simulink model "simulink_traverse"  (R2021b)
settings: Solver=ode45  StartTime=0.0  StopTime=20  RelTol=1e-3
values from neighbouring files (symbols this model uses):
  ts3 = 10^-3    (= 0.001)    [loading_project.m]
libraries: simulink x3
settings Model: Creator=noait  LastModifiedBy=noait

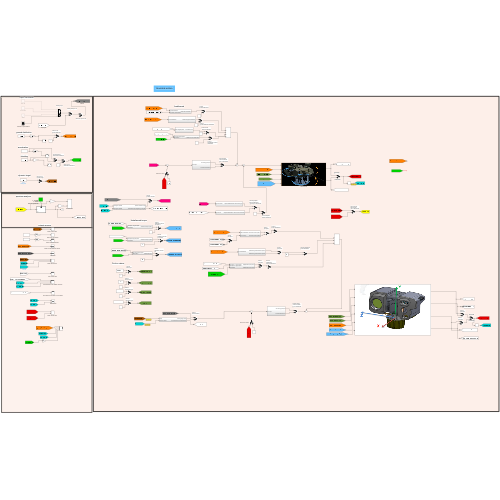
[thumbnail: Simulink's stored preview of the top-level diagram]
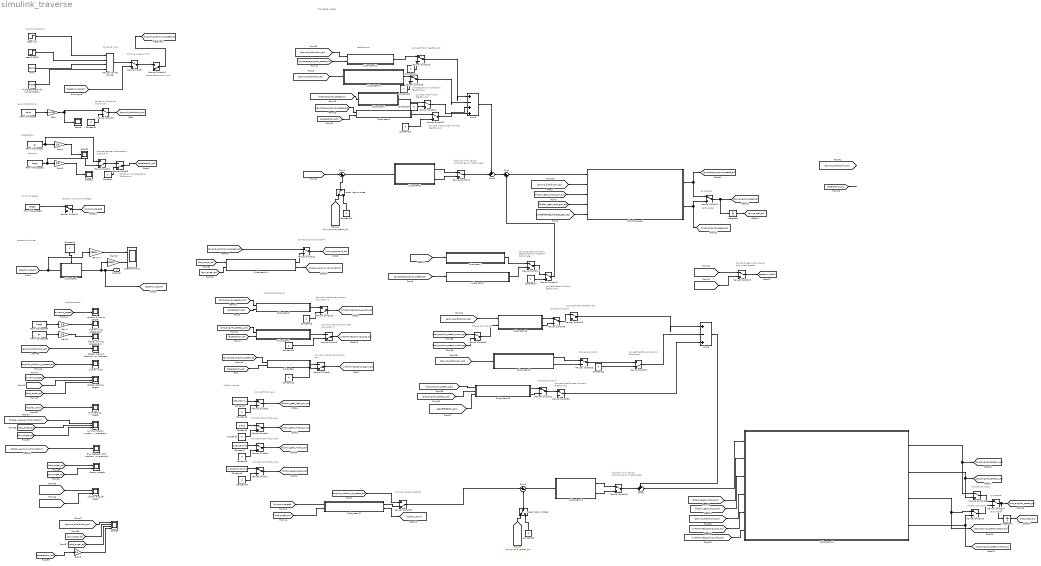
== system simulink_traverse ==
  note: TRAVERSE MODEL
  note: connect motor
      |  friction feedforward
  note: feedforward
  note: spectrum analyzer
  note: dynamic target
  note: acceleration
  note: ground distribution
  note: shooting
  note: input:Time domain
  note: Friction values
  note: Unballanced torque
  note: tachometer
  note: gyroscope
  note: cancel or not
      | synamic target
  note: cancel or not
      | acceleration distribution
  note: choose between
      | acceleration distribution
  note: cancel or not
      | ground distribution
  note: choosing input
  note: chosing sweep or not
  note: disconnect input or not
  note: connect
      | ground distribution feedforward
  note: connect
      | friction feedforward
  note: connect
      | unballanced moment
      | feedforward
  note: chossing setpoint
      | friction feedforward
      |  gyroscope or tachometer
  note: connect setpoint
      | friction feedforward
  note: choose sweep
      | output signal
      |  pod or tachometer
  note: choose
      | pod option
  note: choose
      | pod option
  note: choose
      | pod option
  note: choose
      | pod option
  note: choose
      | pod option
  note: choose
      | pod option
  note: gyroscope
  note: tachometer
  note: chossing which
      |  sensor controller
      | gyro or tachometer
  note: chossing which
      |  sensor controller
      | gyro or tachometer
  note: connect
      | friction gun
  note: connect
      | motor friction-gun
  note: connect
      | motor friction-pod
  note: connect
      | load friction-pod
  note: connect
      | unballance moment
      | gun
  note: connect
      | unballance moment
      | pod option 2
  note: connect
      | unballance moment
      | pod option 1
  note: connect
      | position controller
  note: connect feedforward
      | ground distribution
  note: connect
      | friction feedforward
  note: connect
      | unballanced
      | moment feedforward
  note: connect
      | inertia controller
  note: outputs scopes
  " plant traverse4" : Subsystem
      mask Display: image('C:\Users\noait\OneDrive\Desktop\צילום.png'); % Use "Edit Image" on toolstrip to change.
  " synchronization system stability accuaracy" : Scope  NumInputPorts=3
  Constant : Constant  Value=0  SampleTime=-1
  Constant1 : Constant  OutDataTypeStr=boolean
      settings: AttributesFormatString=1 - START\n0 -STOP\ninternal spectrum
      settings: OpenFcn=|
      | if get_param(gcbh,'value')-48 set_param(gcbh,'value','0','backgroundcolor','red');
      | else set_param(gcbh,'value','1','backgroundcolor','green');
      | end
  Constant{4,6,8,10..20,22} (15 alike) : Constant  Value=0  SampleTime=0
  Constant2 : Constant  Value=0  SampleTime=-1
  Constant3 : Constant  Value=0.021  SampleTime=0
  Constant5 : Constant  Value=1300/(200*1.1)  SampleTime=0
  Constant7 : Constant  Value=0.23125*0.42  SampleTime=0
  Constant9 : Constant  Value=0.23125*0.42*0.5  SampleTime=0
  Error between pod position to gun position1 : Scope
  From Workspace : FromWorkspace  VariableName=trdist  SampleTime=ts3/3  Interpolate=off  ZeroCross=off  OutputAfterFinalValue=Setting to zero
  From Workspace1 : FromWorkspace  VariableName=gy  SampleTime=ts3/3  Interpolate=off  ZeroCross=off  OutputAfterFinalValue=Setting to zero
  From Workspace2 : FromWorkspace  VariableName=firegy  SampleTime=ts3/9  Interpolate=off  ZeroCross=off  OutputAfterFinalValue=Setting to zero
  From Workspace3 : FromWorkspace  VariableName=targetx  SampleTime=5*ts3  Interpolate=off  ZeroCross=off  OutputAfterFinalValue=Setting to zero
  From Workspace4 : FromWorkspace  VariableName=firegz  SampleTime=ts3/9  Interpolate=off  ZeroCross=off  OutputAfterFinalValue=Setting to zero
  From Workspace5 : FromWorkspace  VariableName=gz  SampleTime=ts3/3  Interpolate=off  ZeroCross=off  OutputAfterFinalValue=Setting to zero
  Gain : Gain  Gain=pi/180
  Gain{1..5} (5 alike) : Gain  Gain=9.8
  Gain17 : Gain  Gain=180/pi
  Gain18 : Gain  Gain=180/pi
  Integrator : Integrator  ZeroCross=off
  Integrator1 : Integrator  ZeroCross=off
  Manual Variant Source : simulink/Signal Routing/Manual Variant Source  NumChoices=4  LabelModeActiveChoice=V_4
  Manual Switch{,3..7,11..15,17..26,28..32,34} (27 alike) : ManualSwitch
  Manual Switch{1..2,8..10,16,27,33} (8 alike) : ManualSwitch  CurrentSetting=0
  Pulse Generator for syncronization : DiscretePulseGenerator  PulseType=Time based  Period=10  PulseWidth=50
  Scope : Scope
  Scope1 : Scope
  Scope2 : Scope
  Scope3 : Scope  NumInputPorts=4
  SpectrumInOut : Scope  NumInputPorts=2
  Step 1[A] : Step  SampleTime=0  ZeroCross=off
  Subsystem : Subsystem
  Subsystem1 : Subsystem  mask{GAIN=0.22%2*pi/180%0.5*pi/180, InitFreq=1, TargetTime=500, FreqAtTime=500}
      mask prompts: InitFreq "INITIAL FREQUENCY"; TargetTime "Target Time"; FreqAtTime "Frequency at Time"
  Subsystem10 : Subsystem
  Subsystem11 : Subsystem
      mask Display: image('C:\Users\noait\OneDrive\Desktop\צילום מסך 2024-04-08 195106.png'); % Use "Edit Image" on toolstrip to change.
  Subsystem12 : Subsystem
  Subsystem13 : Subsystem
  Subsystem14 : Subsystem
  Subsystem15 : Subsystem
  Subsystem16 : Subsystem
  Subsystem17 : Subsystem
  Subsystem2 : Subsystem
  Subsystem3 : Subsystem
  Subsystem4 : Subsystem
  Subsystem5 : Subsystem
  Subsystem6 : Subsystem
  Subsystem7 : Subsystem
  Subsystem8 : Subsystem
  Subsystem9 : Subsystem
  Sum : Sum  Inputs=|++
  Sum1 : Sum  Inputs=|+-
  Sum2 : Sum  Inputs=++|
  Sum3 : Sum  Inputs=|+-++
  Sum4 : Sum  Inputs=|+-
  Sum5 : Sum  Inputs=++|
  Sum6 : Sum  Inputs=|+-+
  display angels : Scope  NumInputPorts=2
  display angular speed : Scope  NumInputPorts=2
  display driving acceleration : Scope
  display dynamic target : Scope
  display firing acceleration : Scope
  display ground distribution [rad/sec] : Scope
  display input : Scope
  display tracking target : Scope  NumInputPorts=3
  error tracking target : Scope
  open loop or close : ManualSwitch
  open loop or close1 : ManualSwitch
  ramp : simulink/Sources/Ramp  slope=1  start=0  InitialOutput=0
  step 0.05[A] : Step  After=0.05  SampleTime=0  ZeroCross=off
  Output2 : Outport
  wires:
  Pulse Generator for syncronization/1 -> Manual Variant Source/4
  Manual Switch/1 -> Manual Switch16/1
  Manual Switch2/1 -> [acceleration_az]
  Manual Switch1/1 -> Manual Switch2/1
  From Workspace2/1 -> Manual Switch1/2, Gain2/1
  Manual Switch16/1 -> [angular_position_or_speed_az]
  Constant2/1 -> Manual Switch3/2
  Gain1/1 -> Scope1/1
  Gain/1 -> Manual Switch3/1, Scope/1
  Manual Switch3/1 -> [ground_distribution_az]
  Gain2/1 -> Scope2/1
  Constant/1 -> Manual Switch2/2
  Manual Variant Source/1 -> Manual Switch/1
  Step 1[A]/1 -> Manual Variant Source/1
  From Workspace1/1 -> Manual Switch1/1, Gain1/1
  step 0.05[A]/1 -> Manual Variant Source/2
  ramp/1 -> Manual Variant Source/3
  From Workspace/1 -> Gain/1
  [spectrum_signal] -> Manual Switch/2
  Manual Switch4/1 -> [friction_gear_motor_gun_az]
  Constant6/1 -> Manual Switch5/2
  Manual Switch5/1 -> [friction_gear_load_gun_az]
  Constant10/1 -> Manual Switch7/2
  Constant8/1 -> Manual Switch6/2
  Constant4/1 -> Manual Switch4/2
  Manual Switch7/1 -> [friction_gear_load_pod]
  Manual Switch6/1 -> [friction_gear_motor_pod]
  Constant5/1 -> Manual Switch5/1
  Constant7/1 -> Manual Switch6/1
  Constant9/1 -> Manual Switch7/1
  Constant3/1 -> Manual Switch4/1
  [gyroscope_angular_speed_az] -> Subsystem/1(gyroscope angular speed)
  [acceleration_az] -> Subsystem/2(acceleration)
  [acceleration_az] -> Subsystem2/2(acceleration)
  Subsystem2/1(unballanced torque option2) -> Manual Switch9/1
  Constant11/1 -> Manual Switch8/2
  Subsystem/1(unballanced torque) -> Manual Switch8/1
  Manual Switch10/1 -> [unballanced_torque_pod1_az]
  [acceleration_az] -> Subsystem3/2(acceleration)
  Manual Switch8/1 -> [unballanced_torque_gun_az]
  Manual Switch9/1 -> [unballanced_torque_pod2_az]
  Subsystem3/1(unballanced torque option1) -> Manual Switch10/1
  Constant13/1 -> Manual Switch10/2
  [pod_angular_speed_2_az] -> Subsystem2/1(pod option2 angular speed)
  Constant12/1 -> Manual Switch9/2
  [pod_angular_speed_1_az] -> Subsystem3/1("pod option1  angular speed ")
  [ground_distribution_az] -> " plant traverse4"/2(external distribution)
  [friction_gear_load_gun_az] -> " plant traverse4"/4(load friction az value)
  [friction_gear_motor_gun_az] -> " plant traverse4"/3(motor friction value az)
  [unballanced_torque_gun_az] -> " plant traverse4"/5(unballanced torque az)
  Integrator/1 -> [gun_angel_az]
  Manual Switch12/1 -> Integrator/1, [gun_angular_speed_az]
  " plant traverse4"/1(gun speed gyroscope) -> [gyroscope_angular_speed_az], Manual Switch12/1
  " plant traverse4"/2(motor speed tachometer) -> [motor_angular_speed_az], Manual Switch12/2
  Gain17/1 -> SpectrumInOut/1
  Gain18/1 -> SpectrumInOut/2
  [spectrum_back] -> Gain17/1, Subsystem1/1(Input)
  Subsystem1/1(Output2) -> [spectrum_signal], Output2/1, Gain18/1
  Constant1/1 -> Subsystem1/Enable
  Manual Switch25/1 -> [spectrum_back]
  [gun_angular_speed_az] -> Manual Switch25/1
  [pod_angular_speed_az] -> Manual Switch25/2
  Subsystem5/2(out control tachometer) -> Manual Switch13/2
  Subsystem5/1(out control gyroscope) -> Manual Switch13/1
  Sum1/1 -> Subsystem5/1(error input)
  Constant14/1 -> open loop or close/2
  [gun_angular_speed_az] -> open loop or close/1
  open loop or close/1 -> Sum1/2
  [input_command_az] -> Sum1/1
  Manual Switch11/1 -> [input_command_az]
  Sum/1 -> " plant traverse4"/1(current command traverse)
  Sum2/1 -> Sum/1
  [gyroscope_angular_speed_az] -> Subsystem4/1(gyroscope angular speed)
  [acceleration_az] -> Subsystem4/2(acceleration)
  Manual Switch13/1 -> Sum2/2
  Sum3/1 -> Sum2/1
  Manual Switch21/1 -> Sum3/3
  Subsystem4/1(unballanced torque feedforward) -> Manual Switch21/1
  Constant15/1 -> Manual Switch21/2
  Subsystem7/1(setpoint feedforward for reduce friction gyro) -> Manual Switch17/1
  [gyroscope_angular_speed_az] -> Subsystem8/1(gyro sensor)
  [motor_angular_speed_az] -> Subsystem6/1(motor angular speed)
  Constant16/1 -> Manual Switch14/2
  Subsystem6/1(anti friction motor) -> Manual Switch14/1
  Manual Switch14/1 -> Sum3/4
  Manual Switch17/1 -> Manual Switch18/1
  Subsystem8/1(setpoint feedforward for reduce friction tachometer) -> Manual Switch17/2
  Manual Switch18/1 -> Sum/2
  Constant17/1 -> Manual Switch18/2
  Constant18/1 -> Manual Switch15/2
  Subsystem9/1(feedforward ground distribution) -> Manual Switch15/1
  [ground_distribution_az] -> Subsystem9/1(ground distribution)
  [ground_distribution_az] -> Subsystem10/1(ground distribution)
  Constant19/1 -> Manual Switch19/2
  Subsystem10/1(feedforward load friction) -> Manual Switch19/1
  Manual Switch19/1 -> Sum3/1
  Manual Switch15/1 -> Sum3/2
  [gyroscope_angular_speed_az] -> Subsystem10/2(gyroscope angular speed)
  [friction_gear_motor_pod] -> Subsystem11/2(motor torque value pod)
  [friction_gear_load_pod] -> Subsystem11/3(torque load value pod)
  [ground_distribution_az] -> Subsystem11/4(external distribution)
  [unballanced_torque_pod1_az] -> Subsystem11/5(unballanced torque option1)
  [unballanced_torque_pod2_az] -> Subsystem11/6(unballanced torque option 2)
  Manual Switch23/1 -> Manual Switch24/2
  Subsystem11/3(tachometer motor angular speed option 1) -> [pod_angular_speed_motor1_az], Manual Switch23/1
  Subsystem11/4(tachometer motor angular speed option2) -> [pod_angular_speed_motor2_az], Manual Switch23/2
  Subsystem11/2(gyroscope output option2) -> Manual Switch22/2, [pod_angular_speed_2_az]
  Manual Switch24/1 -> Integrator1/1, [pod_angular_speed_az]
  Integrator1/1 -> [pod_angel_az]
  Subsystem11/1(gyroscope output option 1) -> Manual Switch22/1, [pod_angular_speed_1_az]
  Manual Switch22/1 -> Manual Switch24/1
  [pod_angular_speed_az] -> open loop or close1/1
  Constant20/1 -> open loop or close1/2
  open loop or close1/1 -> Sum4/2
  Sum4/1 -> Subsystem12/1(error input)
  Subsystem12/1(out control gyroscope) -> Manual Switch20/1
  Subsystem12/2(out control tachometer) -> Manual Switch20/2
  Manual Switch20/1 -> Sum5/2
  Sum5/1 -> Subsystem11/1(input current)
  [ground_distribution_az] -> Subsystem13/1(ground distribution)
  Constant22/1 -> Manual Switch27/2
  Manual Switch27/1 -> Sum6/2
  Subsystem13/1(feedforward ground distribution option1) -> Manual Switch26/1
  Subsystem13/2(feedforward ground distribution option2) -> Manual Switch26/2
  Manual Switch26/1 -> Manual Switch27/1
  Sum6/1 -> Sum5/1
  Manual Switch28/1 -> Sum6/1
  Subsystem16/2(unballanced torque option2) -> Manual Switch31/2
  Manual Switch30/1 -> Manual Switch28/1
  [pod_angular_speed_motor2_az] -> Manual Switch29/2
  [pod_angular_speed_2_az] -> Subsystem16/2("pod option2  angular speed ")
  Subsystem15/1(anti friction current option1) -> Manual Switch30/1
  Subsystem15/2(anti friction current option2) -> Manual Switch30/2
  Subsystem16/1(unballanced torque option1) -> Manual Switch31/1
  Manual Switch31/1 -> Manual Switch32/1
  [pod_angular_speed_1_az] -> Subsystem16/1("pod option1  angular speed ")
  [acceleration_az] -> Subsystem16/3(acceleration)
  [ground_distribution_az] -> Subsystem15/1(external distribution)
  [pod_angular_speed_motor1_az] -> Manual Switch29/1
  Manual Switch29/1 -> Subsystem15/2(motor velocity)
  Manual Switch32/1 -> Sum6/3
  [gun_angel_az] -> Subsystem14/2(gun angular position)
  Subsystem14/1(position controller output) -> Manual Switch11/2
  [pod_angel_az] -> Subsystem14/1(pod angular position)
  [angular_position_or_speed_az] -> Manual Switch11/1
  [input_command_az] -> Subsystem7/1(gyro command)
  [pod_angel_az] -> Subsystem17/2(pod gun position)
  Subsystem17/1(error targeting control) -> Manual Switch33/2
  [angular_position_or_speed_az] -> Manual Switch33/1
  Manual Switch33/1 -> Sum4/1
  [acceleration_az] -> ?
  Manual Switch34/1 -> [dynamic_target]
  From Workspace3/1 -> Manual Switch34/1
  [dynamic_target] -> Subsystem17/1(target)
  [gun_angel_az] -> " synchronization system stability accuaracy"/3
  [ground_distribution_az] -> display ground distribution [rad/sec]/1
  [gun_angular_speed_az] -> display angular speed/1
  [gun_angel_az] -> display angels/2
  Gain5/1 -> display driving acceleration/1
  From Workspace5/1 -> Gain5/1
  [dynamic_target] -> display dynamic target/1
  [pod_angel_az] -> display tracking target/3
  [pod_angel_az] -> Scope3/3
  [display_error_synchronization] -> " synchronization system stability accuaracy"/1
  [display_error_synchronization] -> Error between pod position to gun position1/1
  [pod_angel_az] -> display angels/1
  [gun_angel_az] -> display tracking target/2
  [acceleration_az] -> Gain3/1
  From Workspace4/1 -> Gain4/1
  Gain4/1 -> display firing acceleration/1
  [ground_distribution_az] -> Scope3/1
  Gain3/1 -> Scope3/4
  [angular_position_or_speed_az] -> display input/1
  [pod_angular_speed_az] -> display angular speed/2
  [pod_angel_az] -> " synchronization system stability accuaracy"/2
  [gun_angel_az] -> Scope3/2
  [dynamic_target] -> display tracking target/1
  [display_error] -> error tracking target/1
  Subsystem17/2(error between target to pod position) -> [display_error]
  Subsystem14/2(Error between pod angular to gun angular) -> [display_error_synchronization]

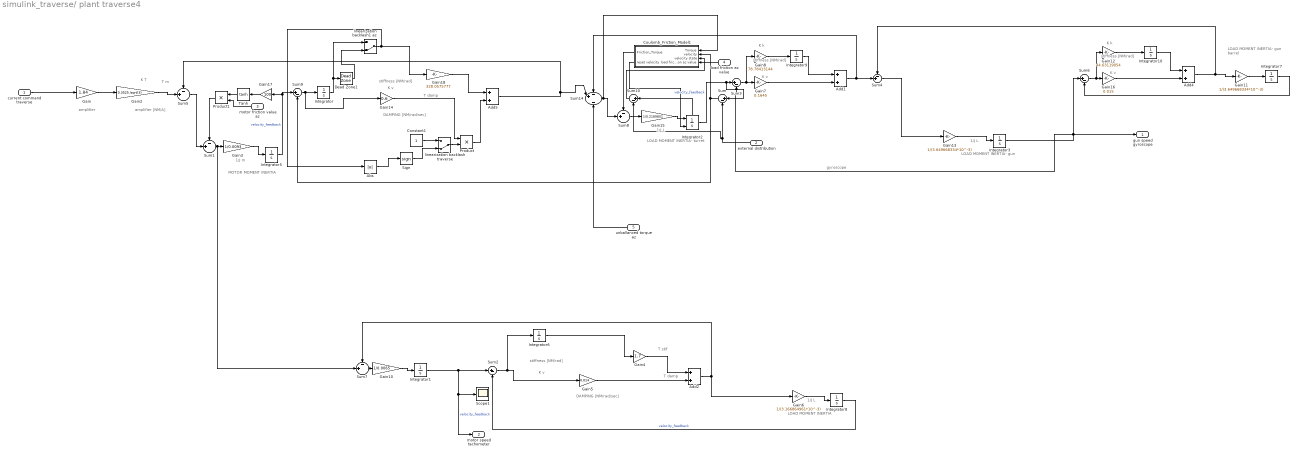
== system simulink_traverse/ plant traverse4 ==
  note: gyroscope
  note: K v
  note: T m
  note: stiffness
      | [NM/rad]
  note: K T
  note: K k
  note: MOTOR
      | MOMENT INERTIA
  note: amplifier
      | [NM/A]
  note: 1/J m
  note: K v
  note: stiffness
      | [NM/rad]
  note: K k
  note: LOAD
      | MOMENT INERTIA- gun
  note: 1/J L
  note: 1/J L
  note: stiffness
      | [NM/rad]
  note: T damp
  note: DAMPING
      | [NM/rad/sec]
  note: LOAD
      | MOMENT INERTIA
  note: K v
  note: T stif
  note: stiffness
      | [NM/rad]
  note: T damp
  note: DAMPING
      | [NM/rad/sec]
  note: LOAD
      | MOMENT INERTIA- turret
  note: K v
  note: 1/J L
  note: LOAD
      | MOMENT INERTIA- gun barrel
  note: amplifier
  current command traverse : Inport
  external distribution : Inport  Port=2
  motor friction value az : Inport  Port=3
  load friction az value : Inport  Port=4
  unballanced torque az : Inport  Port=5
  Abs : Abs
  Add{1..2,4..5} (4 alike) : Sum
  Constant1 : Constant
  Coulomb_Friction_Model1 : Subsystem
  Dead Zone1 : DeadZone  LowerValue=-0.07*10^-3  UpperValue=0.07*10^-3  ZeroCross=off
  Gain : Gain  Gain=1.84
  Gain10 : Gain  Gain=1/0.0065
  Gain11 : Gain  Gain=1/(3.649668334*10^-3)
  Gain12 : Gain  Gain=44.63119054
  Gain13 : Gain  Gain=1/(3.649668334*10^-3)
  Gain14 : Gain  Gain=0.6
  Gain15 : Gain  Gain=1/0.2189801
  Gain16 : Gain  Gain=0.015
  Gain17 : Gain  Gain=100
  Gain18 : Gain  Gain=328.0575777
  Gain2 : Gain  Gain=0.3525 /sqrt(3)
  Gain3 : Gain  Gain=1/0.0093
  Gain4 : Gain  Gain=1.7
  Gain5 : Gain  Gain=0.014
  Gain6 : Gain  Gain=1/(3.166864961*10^-3)
  Gain7 : Gain  Gain=0.1645
  Gain8 : Gain  Gain=78.78413144
  Integrator{,6..7,9..10} (5 alike) : Integrator
  Integrator{1,3,5,8} (4 alike) : Integrator  ZeroCross=off
  Integrator2 : Integrator  ExternalReset=rising  ShowStatePort=on  ZeroCross=off
  Product : Product
  Product1 : Product
  Scope1 : Scope
  Sign : Signum
  Sum{,2..3,6,9..10} (6 alike) : Sum  Inputs=|+-
  Sum1 : Sum  Inputs=-+|  SaturateOnIntegerOverflow=on
  Sum14 : Sum  Inputs=-+|-  SaturateOnIntegerOverflow=on
  Sum4 : Sum  Inputs=-+|
  Sum5 : Sum  Inputs=-+|
  Sum7 : Sum  Inputs=-+|  SaturateOnIntegerOverflow=on
  Sum8 : Sum  Inputs=-+|  SaturateOnIntegerOverflow=on
  Tanh : Trigonometry  Operator=tanh
  linearization backlash traverse : ManualSwitch  CurrentSetting=0
  linearization backlash1 az : ManualSwitch  CurrentSetting=0
  gun speed gyroscope : Outport
  motor speed tachometer : Outport  Port=2
  wires:
  Gain12/1 -> Integrator10/1
  Sum5/1 -> Sum1/2
  Integrator7/1 -> Sum6/2
  Gain/1 -> Gain2/1
  Integrator9/1 -> Add1/1
  Gain3/1 -> Integrator5/1
  Gain16/1 -> Add4/2
  Add1/1 -> Sum4/2, Sum14/1
  Gain6/1 -> Integrator8/1
  Gain14/1 -> Product/1
  Gain2/1 -> Sum5/2
  Sum3/1 -> Gain7/1, Gain8/1
  Gain7/1 -> Add1/2
  Gain10/1 -> Integrator1/1
  Gain11/1 -> Integrator7/1
  Gain8/1 -> Integrator9/1
  Integrator8/1 -> Sum2/2  "velocity_feedback"
  Integrator3/1 -> gun speed gyroscope/1, Sum3/2, Sum6/1
  Sum2/1 -> Integrator6/1, Gain5/1
  Sum4/1 -> Gain13/1
  Add4/1 -> Gain11/1, Sum4/1
  Integrator10/1 -> Add4/1
  Integrator2/1 -> Sum/1, Sum3/1  "velocity_feedback"
  Sum9/1 -> Gain14/1, Integrator/1
  Sum6/1 -> Gain16/1, Gain12/1
  Gain15/1 -> Integrator2/1
  Sum7/1 -> Gain10/1
  Add2/1 -> Gain6/1, Sum7/1
  Sum1/1 -> Sum7/2, Gain3/1
  Integrator5/1 -> Sum9/1, Gain17/1  "velocity_feedback"
  Add5/1 -> Sum5/1, Sum14/2
  Gain13/1 -> Integrator3/1
  Integrator1/1 -> motor speed tachometer/1, Scope1/1, Sum2/1  "velocity_feedback"
  current command traverse/1 -> Gain/1
  Sign/1 -> linearization backlash traverse/2
  Abs/1 -> Sign/1
  linearization backlash traverse/1 -> Product/2
  Constant1/1 -> linearization backlash traverse/1
  Product/1 -> Add5/2
  Dead Zone1/1 -> linearization backlash1 az/2
  Integrator/1 -> linearization backlash1 az/1, Dead Zone1/1
  linearization backlash1 az/1 -> Abs/1, Gain18/1
  Gain18/1 -> Add5/1
  Gain4/1 -> Add2/1
  Gain5/1 -> Add2/2
  Integrator6/1 -> Gain4/1
  Sum8/1 -> Gain15/1
  Sum14/1 -> Coulomb_Friction_Model1/1(Torque), Sum8/2
  Coulomb_Friction_Model1/1(Friction_Torque) -> Sum8/1
  Coulomb_Friction_Model1/2(reset velocity) -> Integrator2/2
  Sum/1 -> Coulomb_Friction_Model1/2(velocity), Sum9/2
  Sum10/1 -> Coulomb_Friction_Model1/3(velocity state)
  external distribution/1 -> Sum10/2, Sum/2
  Integrator2/State -> Sum10/1
  Gain17/1 -> Tanh/1
  Tanh/1 -> Product1/1
  Product1/1 -> Sum1/1
  motor friction value az/1 -> Product1/2
  load friction az value/1 -> Coulomb_Friction_Model1/4(load friction az value)
  unballanced torque az/1 -> Sum14/3

== system simulink_traverse/Subsystem ==
  gyroscope angular speed : Inport
  acceleration : Inport  Port=2
  Cos2 : Trigonometry
  Gain1 : Gain  Gain=4866/200
  Gain2 : Gain  Gain=4866/200
  Integrator : Integrator  ZeroCross=off
  Sum : Sum  Inputs=|++
  unballanced torque : Outport
  wires:
  Integrator/1 -> Cos2/1
  gyroscope angular speed/1 -> Integrator/1
  Cos2/1 -> Gain2/1
  acceleration/1 -> Gain1/1
  Sum/1 -> unballanced torque/1
  Gain1/1 -> Sum/2
  Gain2/1 -> Sum/1

== system simulink_traverse/Subsystem1 ==
  Input : Inport
  Enable : EnablePort  StatesWhenEnabling=reset
  Chirp Signal1 : simulink/Sources/Chirp Signal  f1=1  T=160  f2=160
  Mux2 : Mux  Inputs=2
  Scope2 : Scope
  TSABAD_out_log : Scope
  gain 3 : Gain  Gain=GAIN  SaturateOnIntegerOverflow=on  SampleTime=ts3  OutDataTypeStr=Inherit: Same as input  ParamDataTypeStr=Inherit: Same as input
  Output2 : Outport
  wires:
  gain 3/1 -> Output2/1, Mux2/1
  Input/1 -> Mux2/2
  Mux2/1 -> TSABAD_out_log/1
  Chirp Signal1/1 -> gain 3/1, Scope2/1

== system simulink_traverse/Subsystem10 ==
  ground distribution : Inport
  gyroscope angular speed : Inport  Port=2
  Gain : Gain  Gain=-1
  Gain14 : Gain  Gain=sqrt(3)/0.3525
  Gain15 : Gain  Gain=1300/(200*1.1)
  Gain16 : Gain  Gain=1/1.84
  Gain19 : Gain  Gain=100
  Sum : Sum  Inputs=|++
  Tanh : Trigonometry  Operator=tanh
  Transfer Fcn1 : TransferFcn  Numerator=[0.02219 1.182 1026 1.42*10^4 5.857*10^6]  Denominator="[0.003183 2.538  528.2 3.284*10^4 5.857*10^6]"
  feedforward load friction : Outport
  wires:
  Gain19/1 -> Tanh/1
  Tanh/1 -> Gain15/1
  Gain15/1 -> Gain16/1
  Gain16/1 -> Gain14/1
  Gain14/1 -> feedforward load friction/1
  ground distribution/1 -> Gain/1
  gyroscope angular speed/1 -> Transfer Fcn1/1
  Gain/1 -> Sum/1
  Sum/1 -> Gain19/1
  Transfer Fcn1/1 -> Sum/2

== system simulink_traverse/Subsystem11 ==
  input current : Inport
  motor torque value pod : Inport  Port=2
  torque load value pod : Inport  Port=3
  external distribution : Inport  Port=4
  unballanced torque option1 : Inport  Port=5
  unballanced torque option 2 : Inport  Port=6
  Subsystem : Subsystem
  Subsystem1 : Subsystem
  gyroscope output option 1 : Outport
  gyroscope output option2 : Outport  Port=2
  tachometer motor angular speed option 1 : Outport  Port=3
  tachometer motor angular speed option2 : Outport  Port=4
  wires:
  Subsystem/1(tachometer motor angular speed option1) -> tachometer motor angular speed option 1/1
  Subsystem/2(gyroscope output option1) -> gyroscope output option 1/1
  Subsystem1/1(tachometer motor angular speed option2) -> tachometer motor angular speed option2/1
  Subsystem1/2(gyroscope output option2) -> gyroscope output option2/1
  motor torque value pod/1 -> Subsystem1/2(motor torque value pod), Subsystem/2(motor torque value pod)
  torque load value pod/1 -> Subsystem/3(torque load value pod), Subsystem1/3(torque load value pod)
  external distribution/1 -> Subsystem1/4(external distribution), Subsystem/4(external distribution)
  unballanced torque option1/1 -> Subsystem/5(unballanced torque option1)
  unballanced torque option 2/1 -> Subsystem1/5(unballanced torque option 2)
  input current/1 -> Subsystem1/1(Input current), Subsystem/1(Input current)

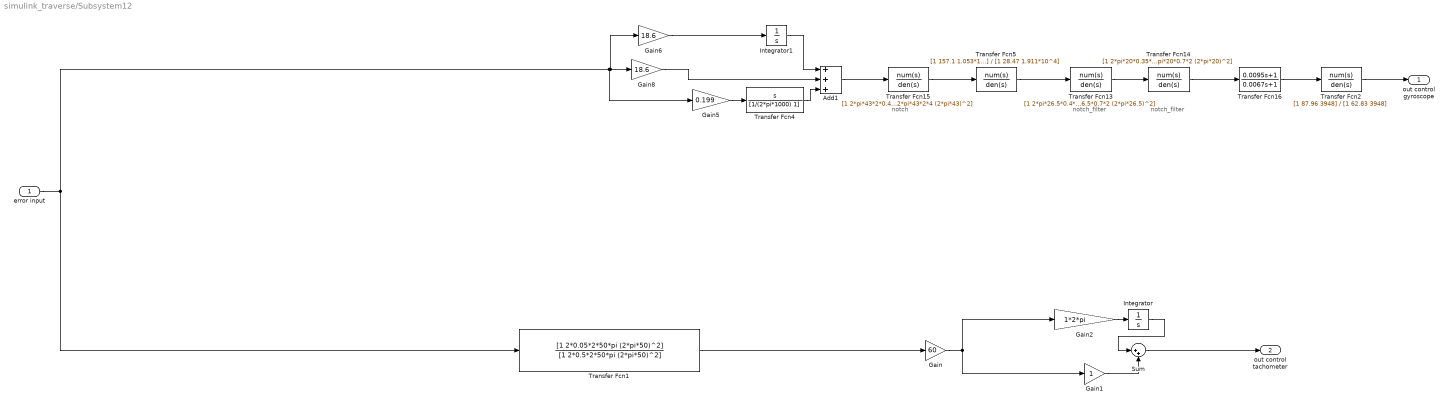
== system simulink_traverse/Subsystem12 ==
  note: notch_filter
  note: notch_filter
  note: notch
  error input : Inport
  Add1 : Sum  Inputs=+++
  Gain : Gain  Gain=60
  Gain1 : Gain
  Gain2 : Gain  Gain=1*2*pi
  Gain5 : Gain  Gain=0.199
  Gain6 : Gain  Gain=18.6
  Gain8 : Gain  Gain=18.6
  Integrator : Integrator
  Integrator1 : Integrator
  Sum : Sum  Inputs=|++
  Transfer Fcn1 : TransferFcn  Numerator=[1 2*0.05*2*50*pi (2*pi*50)^2]  Denominator=[1 2*0.5*2*50*pi (2*pi*50)^2]
  Transfer Fcn13 : TransferFcn  Numerator=[1 2*pi*26.5*0.4*2 (2*pi*26.5)^2]  Denominator=[1 2*pi*26.5*0.7*2 (2*pi*26.5)^2]
  Transfer Fcn14 : TransferFcn  Numerator=[1 2*pi*20*0.35*2 (2*pi*20)^2]  Denominator=[1 2*pi*20*0.7*2 (2*pi*20)^2]
  Transfer Fcn15 : TransferFcn  Numerator="[1 2*pi*43*2*0.4  (2*pi*43)^2]"  Denominator=[1 2*pi*43*2*4 (2*pi*43)^2]
  Transfer Fcn16 : TransferFcn  Numerator=[0.0095 1]  Denominator=[0.0067 1]
  Transfer Fcn2 : TransferFcn  Numerator=[1 87.96 3948]  Denominator=[1 62.83 3948]
  Transfer Fcn4 : TransferFcn  Numerator=[1 0]  Denominator=[1/(2*pi*1000) 1]
  Transfer Fcn5 : TransferFcn  Numerator=[1 157.1 1.053*10^5]  Denominator=[1 28.47 1.911*10^4]
  out control gyroscope : Outport
  out control tachometer : Outport  Port=2
  wires:
  Gain1/1 -> Sum/2
  Gain2/1 -> Integrator/1
  Integrator/1 -> Sum/1
  Gain/1 -> Gain1/1, Gain2/1
  Sum/1 -> out control tachometer/1
  Transfer Fcn1/1 -> Gain/1
  error input/1 -> Transfer Fcn1/1, Gain5/1, Gain6/1, Gain8/1
  Transfer Fcn5/1 -> Transfer Fcn13/1
  Transfer Fcn14/1 -> Transfer Fcn16/1
  Transfer Fcn13/1 -> Transfer Fcn14/1
  Gain5/1 -> Transfer Fcn4/1
  Integrator1/1 -> Add1/1
  Transfer Fcn15/1 -> Transfer Fcn5/1
  Gain6/1 -> Integrator1/1
  Gain8/1 -> Add1/2
  Add1/1 -> Transfer Fcn15/1
  Transfer Fcn4/1 -> Add1/3
  Transfer Fcn16/1 -> Transfer Fcn2/1
  Transfer Fcn2/1 -> out control gyroscope/1

== system simulink_traverse/Subsystem13 ==
  ground distribution : Inport
  Gain1 : Gain  Gain=1/1.4833
  Gain10 : Gain  Gain=1/1.47
  Gain8 : Gain  Gain=0.015
  Gain9 : Gain  Gain=1/1.057
  Transfer Fcn1 : TransferFcn  Numerator=[1 0]  Denominator=[1/(2*pi*1000) 1]
  feedforward ground distribution option1 : Outport
  feedforward ground distribution option2 : Outport  Port=2
  wires:
  Transfer Fcn1/1 -> Gain8/1
  Gain8/1 -> Gain9/1
  Gain9/1 -> Gain1/1, Gain10/1
  ground distribution/1 -> Transfer Fcn1/1
  Gain1/1 -> feedforward ground distribution option2/1
  Gain10/1 -> feedforward ground distribution option1/1

== system simulink_traverse/Subsystem14 ==
  pod angular position : Inport
  gun angular position : Inport  Port=2
  Gain : Gain  Gain=15.5
  Gain1 : Gain
  Gain2 : Gain  Gain=0.8
  Integrator : Integrator  ZeroCross=off
  Sum : Sum  Inputs=|+-
  Sum1 : Sum  Inputs=|+++
  Transfer Fcn : TransferFcn  Numerator=[1 0]  Denominator=[1/(2*pi*100) 1]
  position controller output : Outport
  Error between pod angular to gun angular : Outport  Port=2
  wires:
  pod angular position/1 -> Sum/1
  gun angular position/1 -> Sum/2
  Sum/1 -> Gain2/1, Error between pod angular to gun angular/1, Gain/1
  Sum1/1 -> position controller output/1
  Gain/1 -> Sum1/2, Gain1/1
  Gain1/1 -> Integrator/1
  Integrator/1 -> Sum1/1
  Gain2/1 -> Transfer Fcn/1
  Transfer Fcn/1 -> Sum1/3

== system simulink_traverse/Subsystem15 ==
  external distribution : Inport
  motor velocity : Inport  Port=2
  Gain2 : Gain  Gain=0.23125*0.42*0.5
  Gain21 : Gain  Gain=1/1.057
  Gain23 : Gain  Gain=1/1.483
  Gain3 : Gain  Gain=-1
  Gain4 : Gain  Gain=100
  Gain41 : Gain  Gain=1/1.47
  Gain6 : Gain  Gain=100
  Gain7 : Gain  Gain=0.23125*0.42
  Sum : Sum  Inputs=|++
  Tanh : Trigonometry  Operator=tanh
  Tanh1 : Trigonometry  Operator=tanh
  anti friction current option1 : Outport
  anti friction current option2 : Outport  Port=2
  wires:
  external distribution/1 -> Gain3/1
  Gain3/1 -> Gain4/1
  Gain4/1 -> Tanh/1
  Tanh/1 -> Gain2/1
  Tanh1/1 -> Gain7/1
  Gain6/1 -> Tanh1/1
  motor velocity/1 -> Gain6/1
  Gain7/1 -> Sum/2
  Gain2/1 -> Sum/1
  Sum/1 -> Gain21/1
  Gain41/1 -> anti friction current option1/1
  Gain21/1 -> Gain23/1, Gain41/1
  Gain23/1 -> anti friction current option2/1

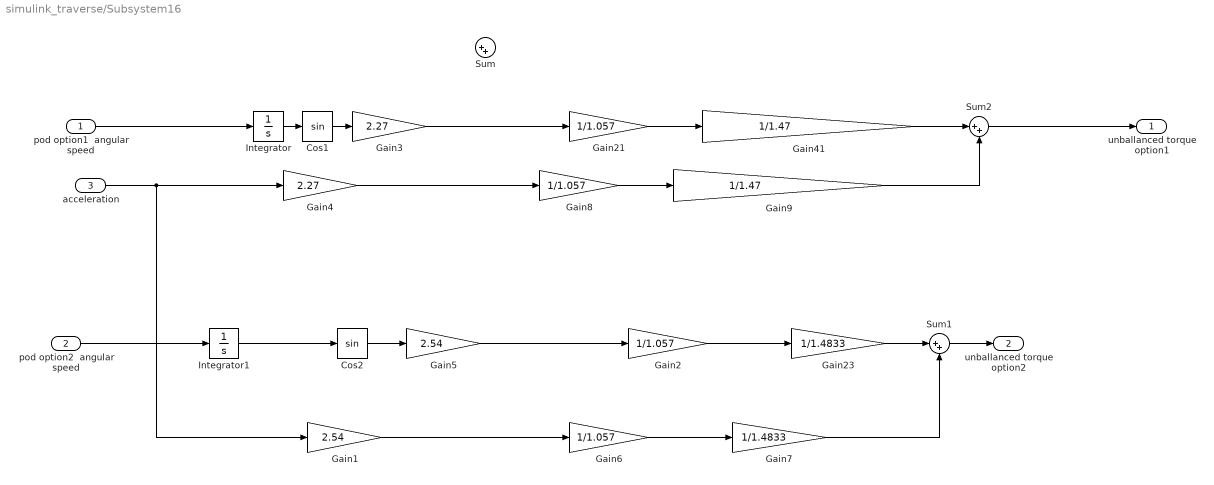
== system simulink_traverse/Subsystem16 ==
  "pod option1  angular speed " : Inport
  "pod option2  angular speed " : Inport  Port=2
  acceleration : Inport  Port=3
  Cos1 : Trigonometry
  Cos2 : Trigonometry
  Gain1 : Gain  Gain=2.54
  Gain{2,6,8,21} (4 alike) : Gain  Gain=1/1.057
  Gain23 : Gain  Gain=1/1.4833
  Gain3 : Gain  Gain=2.27
  Gain4 : Gain  Gain=2.27
  Gain41 : Gain  Gain=1/1.47
  Gain5 : Gain  Gain=2.54
  Gain7 : Gain  Gain=1/1.4833
  Gain9 : Gain  Gain=1/1.47
  Integrator : Integrator  ZeroCross=off
  Integrator1 : Integrator  ZeroCross=off
  Sum : Sum  Inputs=|++
  Sum1 : Sum  Inputs=|++
  Sum2 : Sum  Inputs=|++
  unballanced torque option1 : Outport
  unballanced torque option2 : Outport  Port=2
  wires:
  Integrator/1 -> Cos1/1
  acceleration/1 -> Gain1/1, Gain4/1
  "pod option1  angular speed "/1 -> Integrator/1
  Gain21/1 -> Gain41/1
  Integrator1/1 -> Cos2/1
  "pod option2  angular speed "/1 -> Integrator1/1
  Gain2/1 -> Gain23/1
  Cos1/1 -> Gain3/1
  Gain5/1 -> Gain2/1
  Cos2/1 -> Gain5/1
  Gain23/1 -> Sum1/1
  Sum1/1 -> unballanced torque option2/1
  Gain6/1 -> Gain7/1
  Gain1/1 -> Gain6/1
  Gain7/1 -> Sum1/2
  Gain3/1 -> Gain21/1
  Gain41/1 -> Sum2/1
  Sum2/1 -> unballanced torque option1/1
  Gain8/1 -> Gain9/1
  Gain4/1 -> Gain8/1
  Gain9/1 -> Sum2/2

== system simulink_traverse/Subsystem17 ==
  target : Inport
  pod gun position : Inport  Port=2
  Gain : Gain  Gain=30
  Gain1 : Gain  Gain=30
  Gain2 : Gain  Gain=-0.05
  Integrator2 : Integrator
  Sum : Sum  Inputs=|+-
  Sum1 : Sum  Inputs=|+++
  Transfer Fcn : TransferFcn  Numerator=[1 0]  Denominator=[1/(2*pi*1000) 1]
  error targeting control : Outport
  error between target to pod position : Outport  Port=2
  wires:
  target/1 -> Sum/1
  pod gun position/1 -> Gain2/1, Sum/2
  Integrator2/1 -> Sum1/1
  Gain/1 -> Integrator2/1
  Gain2/1 -> Transfer Fcn/1
  Transfer Fcn/1 -> Sum1/3
  Gain1/1 -> Sum1/2
  Sum1/1 -> error targeting control/1
  Sum/1 -> error between target to pod position/1, Gain/1, Gain1/1

== system simulink_traverse/Subsystem2 ==
  pod option2 angular speed : Inport
  acceleration : Inport  Port=2
  Cos1 : Trigonometry
  Gain1 : Gain  Gain=2.54
  Gain3 : Gain  Gain=2.54
  Integrator : Integrator  ZeroCross=off
  Sum : Sum  Inputs=|++
  unballanced torque option2 : Outport
  wires:
  Cos1/1 -> Gain3/1
  pod option2 angular speed/1 -> Integrator/1
  Integrator/1 -> Cos1/1
  Gain3/1 -> Sum/1
  Sum/1 -> unballanced torque option2/1
  acceleration/1 -> Gain1/1
  Gain1/1 -> Sum/2

== system simulink_traverse/Subsystem3 ==
  "pod option1  angular speed " : Inport
  acceleration : Inport  Port=2
  Cos1 : Trigonometry
  Gain1 : Gain  Gain=2.27
  Gain3 : Gain  Gain=2.27
  Integrator : Integrator  ZeroCross=off
  Sum : Sum  Inputs=|++
  unballanced torque option1 : Outport
  wires:
  Cos1/1 -> Gain3/1
  Integrator/1 -> Cos1/1
  "pod option1  angular speed "/1 -> Integrator/1
  acceleration/1 -> Gain1/1
  Gain1/1 -> Sum/2
  Gain3/1 -> Sum/1
  Sum/1 -> unballanced torque option1/1

== system simulink_traverse/Subsystem4 ==
  gyroscope angular speed : Inport
  acceleration : Inport  Port=2
  Cos2 : Trigonometry
  Gain1 : Gain  Gain=4866/200
  Gain2 : Gain  Gain=4866/200
  Gain6 : Gain  Gain=1/1.84
  Gain7 : Gain  Gain=sqrt(3)/0.3525
  Integrator : Integrator  ZeroCross=off
  Sum : Sum  Inputs=|++
  Transfer Fcn : TransferFcn  Numerator=[0.04139 2.67 1460]  Denominator=[1.5292*10^-5 1.078 546.8]
  unballanced torque feedforward : Outport
  wires:
  Integrator/1 -> Cos2/1
  gyroscope angular speed/1 -> Integrator/1
  Cos2/1 -> Gain2/1
  acceleration/1 -> Gain1/1
  Gain6/1 -> Gain7/1
  Sum/1 -> unballanced torque feedforward/1
  Gain2/1 -> Gain6/1
  Gain7/1 -> Sum/1
  Gain1/1 -> Transfer Fcn/1
  Transfer Fcn/1 -> Sum/2

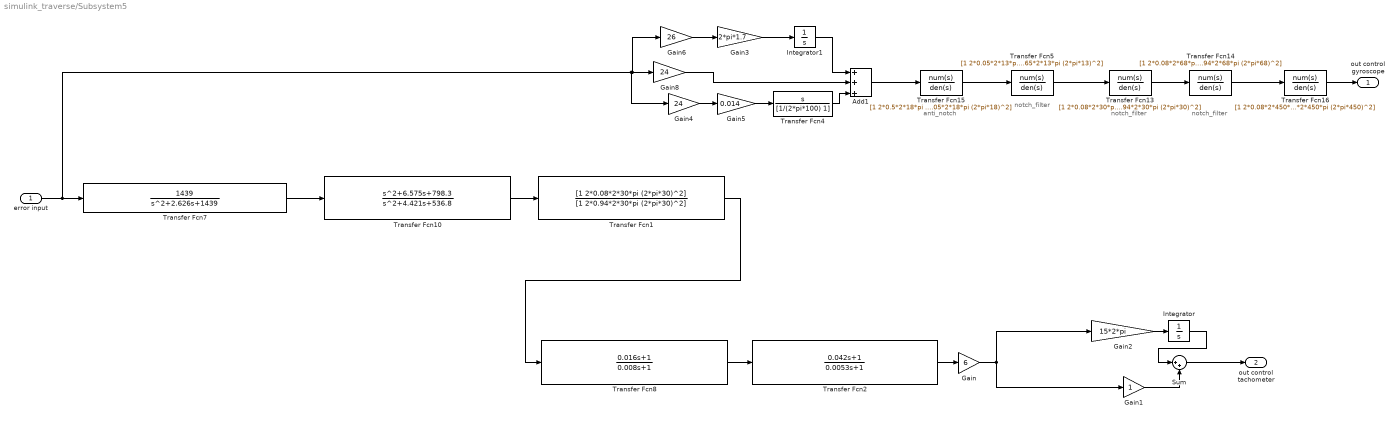
== system simulink_traverse/Subsystem5 ==
  note: notch_filter
  note: notch_filter
  note: notch_filter
  note: anti_notch
  error input : Inport
  Add1 : Sum  Inputs=+++
  Gain : Gain  Gain=6
  Gain1 : Gain
  Gain2 : Gain  Gain=15*2*pi
  Gain3 : Gain  Gain=2*pi*1.7
  Gain4 : Gain  Gain=24
  Gain5 : Gain  Gain=0.014
  Gain6 : Gain  Gain=26
  Gain8 : Gain  Gain=24
  Integrator : Integrator
  Integrator1 : Integrator
  Sum : Sum  Inputs=|++
  Transfer Fcn1 : TransferFcn  Numerator=[1 2*0.08*2*30*pi (2*pi*30)^2]  Denominator=[1 2*0.94*2*30*pi (2*pi*30)^2]
  Transfer Fcn10 : TransferFcn  Numerator=[1 6.575 798.3]  Denominator=[1 4.421 536.8]
  Transfer Fcn13 : TransferFcn  Numerator=[1 2*0.08*2*30*pi (2*pi*30)^2]  Denominator=[1 2*0.94*2*30*pi (2*pi*30)^2]
  Transfer Fcn14 : TransferFcn  Numerator=[1 2*0.08*2*68*pi (2*pi*68)^2]  Denominator=[1 2*0.94*2*68*pi (2*pi*68)^2]
  Transfer Fcn15 : TransferFcn  Numerator=[1 2*0.5*2*18*pi (2*pi*18)^2]  Denominator=[1 2*0.05*2*18*pi (2*pi*18)^2]
  Transfer Fcn16 : TransferFcn  Numerator=[1 2*0.08*2*450*pi (2*pi*450)^2]  Denominator=[1 2*0.94*2*450*pi (2*pi*450)^2]
  Transfer Fcn2 : TransferFcn  Numerator=[0.042 1]  Denominator=[0.0053 1]
  Transfer Fcn4 : TransferFcn  Numerator=[1 0]  Denominator=[1/(2*pi*100) 1]
  Transfer Fcn5 : TransferFcn  Numerator=[1 2*0.05*2*13*pi (2*pi*13)^2]  Denominator=[1 2*0.65*2*13*pi (2*pi*13)^2]
  Transfer Fcn7 : TransferFcn  Numerator=[1439]  Denominator=[1 2.626 1439]
  Transfer Fcn8 : TransferFcn  Numerator=[0.016 1]  Denominator=[0.008 1]
  out control gyroscope : Outport
  out control tachometer : Outport  Port=2
  wires:
  Gain1/1 -> Sum/2
  Transfer Fcn10/1 -> Transfer Fcn1/1
  Transfer Fcn1/1 -> Transfer Fcn8/1
  Gain2/1 -> Integrator/1
  Integrator/1 -> Sum/1
  Gain/1 -> Gain1/1, Gain2/1
  Sum/1 -> out control tachometer/1
  Transfer Fcn7/1 -> Transfer Fcn10/1
  Transfer Fcn8/1 -> Transfer Fcn2/1
  Transfer Fcn2/1 -> Gain/1
  Gain4/1 -> Gain5/1
  Transfer Fcn5/1 -> Transfer Fcn13/1
  error input/1 -> Gain4/1, Gain6/1, Gain8/1, Transfer Fcn7/1
  Transfer Fcn16/1 -> out control gyroscope/1
  Transfer Fcn14/1 -> Transfer Fcn16/1
  Transfer Fcn13/1 -> Transfer Fcn14/1
  Gain5/1 -> Transfer Fcn4/1
  Integrator1/1 -> Add1/1
  Transfer Fcn15/1 -> Transfer Fcn5/1
  Gain3/1 -> Integrator1/1
  Gain8/1 -> Add1/2
  Add1/1 -> Transfer Fcn15/1
  Gain6/1 -> Gain3/1
  Transfer Fcn4/1 -> Add1/3

== system simulink_traverse/Subsystem6 ==
  motor angular speed : Inport
  Gain3 : Gain  Gain=100
  Gain4 : Gain  Gain=0.021
  Gain6 : Gain  Gain=1/1.84
  Gain7 : Gain  Gain=sqrt(3)/0.3525
  Tanh : Trigonometry  Operator=tanh
  Transfer Fcn : TransferFcn  Numerator=[0.6989 4.595 558]  Denominator=[1 4.421 536.8]
  anti friction motor : Outport
  wires:
  Transfer Fcn/1 -> Gain3/1
  Tanh/1 -> Gain4/1
  Gain3/1 -> Tanh/1
  Gain6/1 -> Gain7/1
  Gain4/1 -> Gain6/1
  motor angular speed/1 -> Transfer Fcn/1
  Gain7/1 -> anti friction motor/1

== system simulink_traverse/Subsystem7 ==
  gyro command : Inport
  Gain : Gain  Gain=100
  Gain4 : Gain  Gain=1300/(200*1.1)
  Tanh : Trigonometry  Operator=tanh
  Transfer Fcn1 : TransferFcn  Numerator=[0.04139 2.26 1460]  Denominator=[0.0001592 1.078 546.8]
  Transfer Fcn2 : TransferFcn  Numerator=[0.02219 1.182 1026 1.42*10^4 5.857*10^6]  Denominator="[0.003183 2.538  528.2 3.284*10^4 5.857*10^6]"
  setpoint feedforward for reduce friction gyro : Outport
  wires:
  Gain/1 -> Tanh/1
  Transfer Fcn1/1 -> setpoint feedforward for reduce friction gyro/1
  Gain4/1 -> Transfer Fcn1/1
  Tanh/1 -> Gain4/1
  Transfer Fcn2/1 -> Gain/1
  gyro command/1 -> Transfer Fcn2/1

== system simulink_traverse/Subsystem8 ==
  gyro sensor : Inport
  Gain : Gain  Gain=100
  Gain1 : Gain  Gain=1300/(200*1.1)
  Tanh : Trigonometry  Operator=tanh
  Transfer Fcn : TransferFcn  Numerator=[7.317 4391 5.515*10^5 1.896*10^8 4.492*10^9 1.056*10^12]  Denominator=[1 56.78 4.824*10^4 8.677*10^5 3.438*10^8 1.682*10^9 3.955*10^11]
  Transfer Fcn1 : TransferFcn  Numerator=[0.02219 1.182 1026 1.42*10^4 5.857*10^6]  Denominator=[0.003183 2.538 528.2 3.284*10^4 5.857*10^6]
  setpoint feedforward for reduce friction tachometer : Outport
  wires:
  Gain/1 -> Tanh/1
  Tanh/1 -> Gain1/1
  Gain1/1 -> Transfer Fcn/1
  Transfer Fcn/1 -> setpoint feedforward for reduce friction tachometer/1
  Transfer Fcn1/1 -> Gain/1
  gyro sensor/1 -> Transfer Fcn1/1

== system simulink_traverse/Subsystem9 ==
  ground distribution : Inport
  Gain10 : Gain  Gain=sqrt(3)/0.3525
  Gain8 : Gain  Gain=0.0093
  Gain9 : Gain  Gain=1/1.84
  Transfer Fcn1 : TransferFcn  Numerator=[1 0]  Denominator=[1/(2*pi*100) 1]
  feedforward ground distribution : Outport
  wires:
  Transfer Fcn1/1 -> Gain8/1
  Gain8/1 -> Gain9/1
  Gain9/1 -> Gain10/1
  ground distribution/1 -> Transfer Fcn1/1
  Gain10/1 -> feedforward ground distribution/1

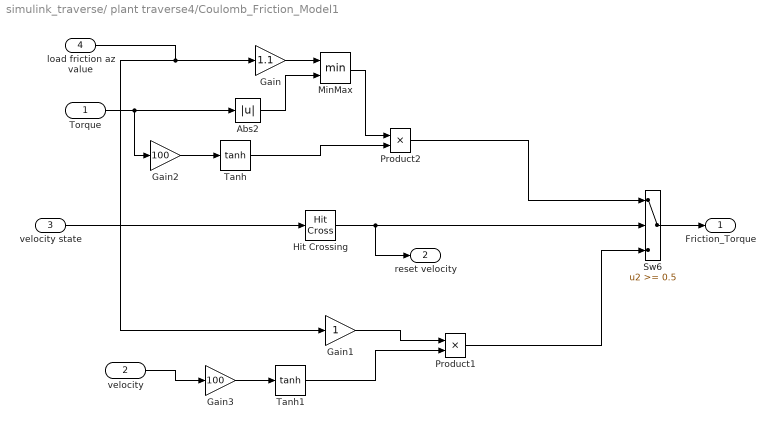
== system simulink_traverse/ plant traverse4/Coulomb_Friction_Model1 ==
  Torque : Inport
  velocity : Inport  Port=2
  velocity state : Inport  Port=3
  load friction az value : Inport  Port=4
  Abs2 : Abs  ZeroCross=off
  Gain : Gain  Gain=1.1
  Gain1 : Gain
  Gain2 : Gain  Gain=100
  Gain3 : Gain  Gain=100
  Hit Crossing : HitCross  ZeroCross=off
  MinMax : MinMax  Inputs=2
  Product1 : Product  RndMeth=Zero
  Product2 : Product  RndMeth=Zero
  Sw6 : Switch  Threshold=0.5  ZeroCross=off  SaturateOnIntegerOverflow=on  InputSameDT=on
  Tanh : Trigonometry  Operator=tanh
  Tanh1 : Trigonometry  Operator=tanh
  Friction_Torque : Outport
  reset velocity : Outport  Port=2
  wires:
  Torque/1 -> Gain2/1, Abs2/1
  Hit Crossing/1 -> reset velocity/1, Sw6/2
  Abs2/1 -> MinMax/2
  MinMax/1 -> Product2/1
  Product2/1 -> Sw6/1
  Product1/1 -> Sw6/3
  velocity state/1 -> Hit Crossing/1
  Gain/1 -> MinMax/1
  Gain1/1 -> Product1/1
  Gain2/1 -> Tanh/1
  Tanh/1 -> Product2/2
  Gain3/1 -> Tanh1/1
  Tanh1/1 -> Product1/2
  velocity/1 -> Gain3/1
  load friction az value/1 -> Gain/1, Gain1/1
  Sw6/1 -> Friction_Torque/1

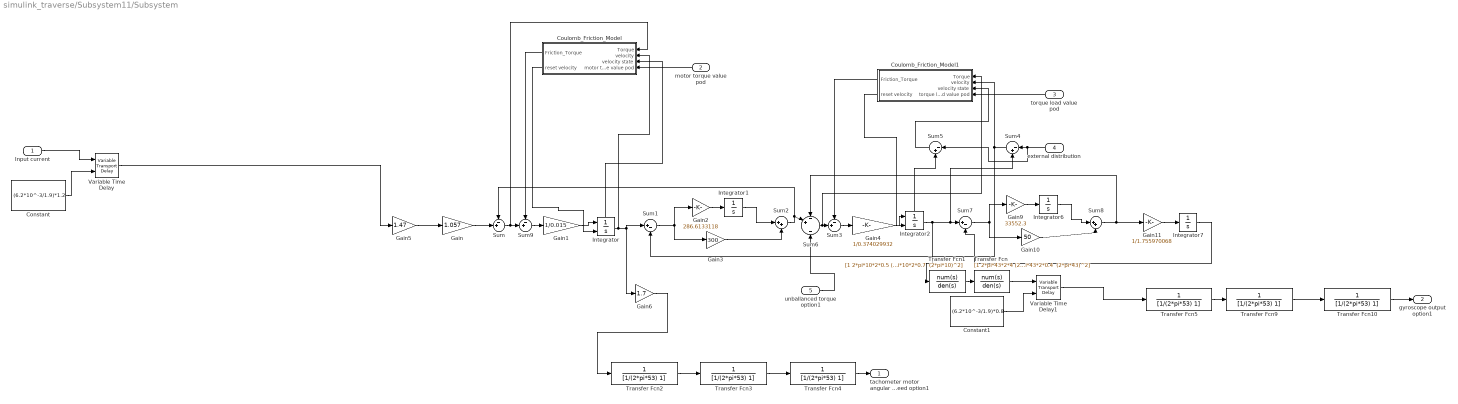
== system simulink_traverse/Subsystem11/Subsystem ==
  Input current : Inport
  motor torque value pod : Inport  Port=2
  torque load value pod : Inport  Port=3
  external distribution : Inport  Port=4
  unballanced torque option1 : Inport  Port=5
  Constant : Constant  Value=(6.2*10^-3/1.9)*1.2  SampleTime=-1
  Constant1 : Constant  Value=(6.2*10^-3/1.9)*0.8  SampleTime=-1
  Coulomb_Friction_Model : Subsystem
  Coulomb_Friction_Model1 : Subsystem
  Gain : Gain  Gain=1.057
  Gain1 : Gain  Gain=1/0.015
  Gain10 : Gain  Gain=50
  Gain11 : Gain  Gain=1/1.755970068
  Gain2 : Gain  Gain=286.6133118
  Gain3 : Gain  Gain=300
  Gain4 : Gain  Gain=1/0.374029932
  Gain5 : Gain  Gain=1.47
  Gain6 : Gain  Gain=1.7
  Gain9 : Gain  Gain=33552.3
  Integrator : Integrator  ExternalReset=rising  ShowStatePort=on  ZeroCross=off
  Integrator1 : Integrator
  Integrator2 : Integrator  ExternalReset=rising  ShowStatePort=on  ZeroCross=off
  Integrator6 : Integrator
  Integrator7 : Integrator
  Sum : Sum  Inputs=-+|
  Sum1 : Sum  Inputs=|+-
  Sum2 : Sum  Inputs=|++
  Sum3 : Sum  Inputs=-+|
  Sum4 : Sum  Inputs=|-+
  Sum5 : Sum  Inputs=|-+
  Sum6 : Sum  Inputs=-+|-
  Sum7 : Sum  Inputs=|+-
  Sum8 : Sum  Inputs=|++
  Sum9 : Sum  Inputs=-+|
  Transfer Fcn : TransferFcn  Numerator=[1 2*pi*43*2*4 (2*pi*43)^2]  Denominator="[1 2*pi*43*2*0.4  (2*pi*43)^2]"
  Transfer Fcn1 : TransferFcn  Numerator=[1 2*pi*10*2*0.5 (2*pi*10)^2]  Denominator="[1 2*pi*10*2*0.7  (2*pi*10)^2]"
  Transfer Fcn{2..5,9..10} (6 alike) : TransferFcn  Denominator=[1/(2*pi*53) 1]
  Variable Time Delay : VariableTransportDelay  MaximumDelay=10  TransDelayFeedthrough=on
  Variable Time Delay1 : VariableTransportDelay  MaximumDelay=10  TransDelayFeedthrough=on
  tachometer motor angular speed option1 : Outport
  gyroscope output option1 : Outport  Port=2
  wires:
  Sum1/1 -> Gain3/1, Gain2/1
  Transfer Fcn/1 -> Variable Time Delay1/1
  Constant1/1 -> Variable Time Delay1/2
  Variable Time Delay/1 -> Gain5/1
  Gain1/1 -> Integrator/1
  Sum8/1 -> Gain11/1, Sum6/1
  Gain11/1 -> Integrator7/1
  Input current/1 -> Variable Time Delay/1
  Integrator2/1 -> Transfer Fcn1/1, Sum4/2, Sum7/1
  Sum2/1 -> Sum6/2, Sum/1
  Integrator7/1 -> Sum7/2
  Gain10/1 -> Sum8/2
  Constant/1 -> Variable Time Delay/2
  Gain2/1 -> Integrator1/1
  Gain5/1 -> Gain/1
  Gain/1 -> Sum/2
  Gain3/1 -> Sum2/2
  Gain4/1 -> Integrator2/1
  Gain9/1 -> Integrator6/1
  Integrator6/1 -> Sum8/1
  Sum7/1 -> Gain10/1, Gain9/1
  Integrator1/1 -> Sum2/1
  motor torque value pod/1 -> Coulomb_Friction_Model/4(motor torque value pod)
  Coulomb_Friction_Model/2(reset velocity) -> Integrator/2
  Sum/1 -> Coulomb_Friction_Model/1(Torque), Sum9/2
  Coulomb_Friction_Model/1(Friction_Torque) -> Sum9/1
  Integrator/1 -> Coulomb_Friction_Model/2(velocity), Sum1/1, Gain6/1
  Integrator/State -> Coulomb_Friction_Model/3(velocity state)
  Coulomb_Friction_Model1/2(reset velocity) -> Integrator2/2
  torque load value pod/1 -> Coulomb_Friction_Model1/4(torque load value pod)
  Sum6/1 -> Coulomb_Friction_Model1/1(Torque), Sum3/2
  Sum3/1 -> Gain4/1
  Coulomb_Friction_Model1/1(Friction_Torque) -> Sum3/1
  external distribution/1 -> Sum5/1, Sum4/1
  Sum4/1 -> Sum1/2, Coulomb_Friction_Model1/2(velocity)
  Integrator2/State -> Sum5/2
  Sum5/1 -> Coulomb_Friction_Model1/3(velocity state)
  unballanced torque option1/1 -> Sum6/3
  Sum9/1 -> Gain1/1
  Transfer Fcn1/1 -> Transfer Fcn/1
  Transfer Fcn2/1 -> Transfer Fcn3/1
  Transfer Fcn3/1 -> Transfer Fcn4/1
  Transfer Fcn4/1 -> tachometer motor angular speed option1/1
  Gain6/1 -> Transfer Fcn2/1
  Transfer Fcn5/1 -> Transfer Fcn9/1
  Transfer Fcn9/1 -> Transfer Fcn10/1
  Transfer Fcn10/1 -> gyroscope output option1/1
  Variable Time Delay1/1 -> Transfer Fcn5/1

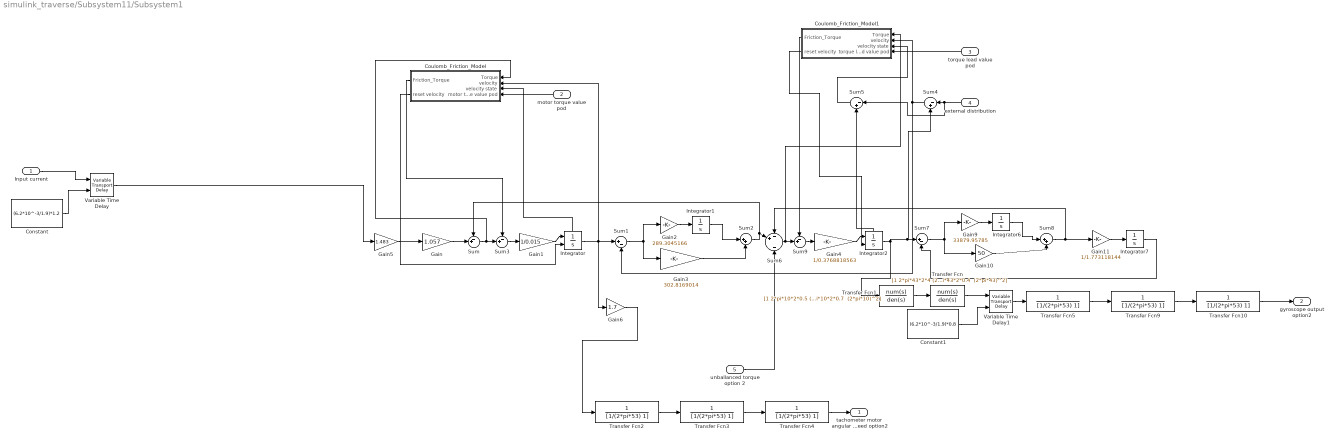
== system simulink_traverse/Subsystem11/Subsystem1 ==
  Input current : Inport
  motor torque value pod : Inport  Port=2
  torque load value pod : Inport  Port=3
  external distribution : Inport  Port=4
  unballanced torque option 2 : Inport  Port=5
  Constant : Constant  Value=(6.2*10^-3/1.9)*1.2  SampleTime=-1
  Constant1 : Constant  Value=(6.2*10^-3/1.9)*0.8  SampleTime=-1
  Coulomb_Friction_Model : Subsystem
  Coulomb_Friction_Model1 : Subsystem
  Gain : Gain  Gain=1.057
  Gain1 : Gain  Gain=1/0.015
  Gain10 : Gain  Gain=50
  Gain11 : Gain  Gain=1/1.773118144
  Gain2 : Gain  Gain=289.3045166
  Gain3 : Gain  Gain=302.8169014
  Gain4 : Gain  Gain=1/0.3768818563
  Gain5 : Gain  Gain=1.483
  Gain6 : Gain  Gain=1.7
  Gain9 : Gain  Gain=33879.95785
  Integrator : Integrator  ExternalReset=rising  ShowStatePort=on  ZeroCross=off
  Integrator1 : Integrator
  Integrator2 : Integrator  ExternalReset=rising  ShowStatePort=on  ZeroCross=off
  Integrator6 : Integrator
  Integrator7 : Integrator
  Sum : Sum  Inputs=-+|
  Sum1 : Sum  Inputs=|+-
  Sum2 : Sum  Inputs=|++
  Sum3 : Sum  Inputs=-+|
  Sum4 : Sum  Inputs=|-+
  Sum5 : Sum  Inputs=|-+
  Sum6 : Sum  Inputs=-+|-
  Sum7 : Sum  Inputs=|+-
  Sum8 : Sum  Inputs=|++
  Sum9 : Sum  Inputs=-+|
  Transfer Fcn : TransferFcn  Numerator=[1 2*pi*43*2*4 (2*pi*43)^2]  Denominator="[1 2*pi*43*2*0.4  (2*pi*43)^2]"
  Transfer Fcn1 : TransferFcn  Numerator=[1 2*pi*10*2*0.5 (2*pi*10)^2]  Denominator="[1 2*pi*10*2*0.7  (2*pi*10)^2]"
  Transfer Fcn{2..5,9..10} (6 alike) : TransferFcn  Denominator=[1/(2*pi*53) 1]
  Variable Time Delay : VariableTransportDelay  MaximumDelay=10  TransDelayFeedthrough=on
  Variable Time Delay1 : VariableTransportDelay  MaximumDelay=10  TransDelayFeedthrough=on
  tachometer motor angular speed option2 : Outport
  gyroscope output option2 : Outport  Port=2
  wires:
  Sum1/1 -> Gain3/1, Gain2/1
  Transfer Fcn/1 -> Variable Time Delay1/1
  Constant1/1 -> Variable Time Delay1/2
  Variable Time Delay/1 -> Gain5/1
  Gain1/1 -> Integrator/1
  Sum8/1 -> Gain11/1, Sum6/1
  Gain11/1 -> Integrator7/1
  Input current/1 -> Variable Time Delay/1
  Integrator2/1 -> Sum4/2, Sum7/1, Transfer Fcn1/1
  Sum2/1 -> Sum6/2, Sum/1
  Integrator7/1 -> Sum7/2
  Gain10/1 -> Sum8/2
  Constant/1 -> Variable Time Delay/2
  Gain2/1 -> Integrator1/1
  Gain5/1 -> Gain/1
  Gain/1 -> Sum/2
  Gain3/1 -> Sum2/2
  Gain4/1 -> Integrator2/1
  Gain9/1 -> Integrator6/1
  Integrator6/1 -> Sum8/1
  Sum7/1 -> Gain10/1, Gain9/1
  Integrator1/1 -> Sum2/1
  Coulomb_Friction_Model/1(Friction_Torque) -> Sum3/1
  Sum/1 -> Coulomb_Friction_Model/1(Torque), Sum3/2
  Integrator/State -> Coulomb_Friction_Model/3(velocity state)
  Integrator/1 -> Coulomb_Friction_Model/2(velocity), Gain6/1, Sum1/1
  Coulomb_Friction_Model/2(reset velocity) -> Integrator/2
  motor torque value pod/1 -> Coulomb_Friction_Model/4(motor torque value pod)
  Coulomb_Friction_Model1/1(Friction_Torque) -> Sum9/1
  Coulomb_Friction_Model1/2(reset velocity) -> Integrator2/2
  external distribution/1 -> Sum5/1, Sum4/1
  Sum6/1 -> Coulomb_Friction_Model1/1(Torque), Sum9/2
  torque load value pod/1 -> Coulomb_Friction_Model1/4(torque load value pod)
  Sum4/1 -> Sum1/2, Coulomb_Friction_Model1/2(velocity)
  Sum5/1 -> Coulomb_Friction_Model1/3(velocity state)
  Sum3/1 -> Gain1/1
  Sum9/1 -> Gain4/1
  Integrator2/State -> Sum5/2
  unballanced torque option 2/1 -> Sum6/3
  Transfer Fcn1/1 -> Transfer Fcn/1
  Transfer Fcn2/1 -> Transfer Fcn3/1
  Transfer Fcn3/1 -> Transfer Fcn4/1
  Transfer Fcn4/1 -> tachometer motor angular speed option2/1
  Gain6/1 -> Transfer Fcn2/1
  Transfer Fcn5/1 -> Transfer Fcn9/1
  Transfer Fcn9/1 -> Transfer Fcn10/1
  Variable Time Delay1/1 -> Transfer Fcn5/1
  Transfer Fcn10/1 -> gyroscope output option2/1

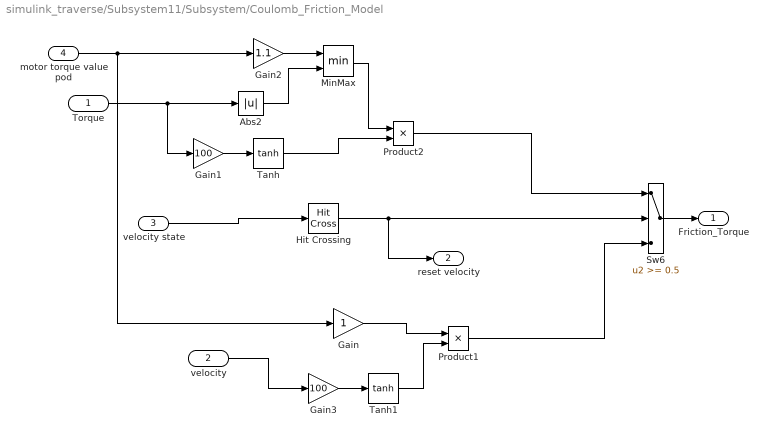
== system simulink_traverse/Subsystem11/Subsystem/Coulomb_Friction_Model ==
  Torque : Inport
  velocity : Inport  Port=2
  velocity state : Inport  Port=3
  motor torque value pod : Inport  Port=4
  Abs2 : Abs  ZeroCross=off
  Gain : Gain
  Gain1 : Gain  Gain=100
  Gain2 : Gain  Gain=1.1
  Gain3 : Gain  Gain=100
  Hit Crossing : HitCross  ZeroCross=off
  MinMax : MinMax  Inputs=2
  Product1 : Product  RndMeth=Zero
  Product2 : Product  RndMeth=Zero
  Sw6 : Switch  Threshold=0.5  ZeroCross=off  SaturateOnIntegerOverflow=on  InputSameDT=on
  Tanh : Trigonometry  Operator=tanh
  Tanh1 : Trigonometry  Operator=tanh
  Friction_Torque : Outport
  reset velocity : Outport  Port=2
  wires:
  Torque/1 -> Gain1/1, Abs2/1
  Hit Crossing/1 -> reset velocity/1, Sw6/2
  Abs2/1 -> MinMax/2
  MinMax/1 -> Product2/1
  Product2/1 -> Sw6/1
  Product1/1 -> Sw6/3
  Gain2/1 -> MinMax/1
  velocity state/1 -> Hit Crossing/1
  Gain/1 -> Product1/1
  Gain1/1 -> Tanh/1
  Gain3/1 -> Tanh1/1
  Tanh/1 -> Product2/2
  Tanh1/1 -> Product1/2
  velocity/1 -> Gain3/1
  motor torque value pod/1 -> Gain2/1, Gain/1
  Sw6/1 -> Friction_Torque/1

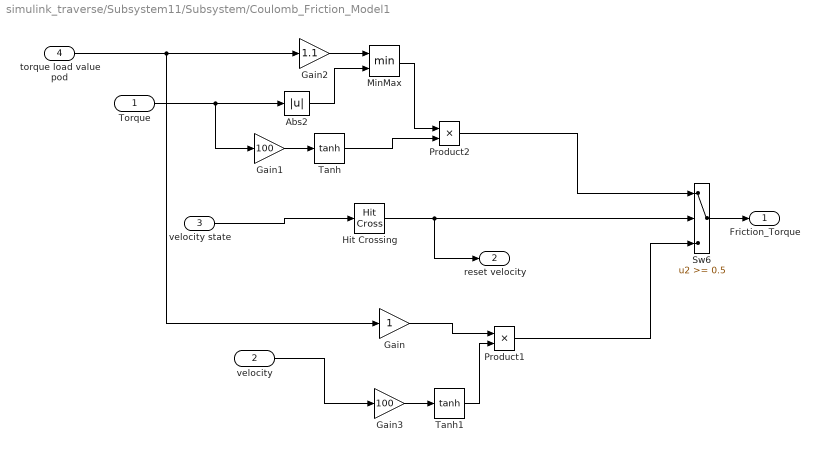
== system simulink_traverse/Subsystem11/Subsystem/Coulomb_Friction_Model1 ==
  Torque : Inport
  velocity : Inport  Port=2
  velocity state : Inport  Port=3
  torque load value pod : Inport  Port=4
  Abs2 : Abs  ZeroCross=off
  Gain : Gain
  Gain1 : Gain  Gain=100
  Gain2 : Gain  Gain=1.1
  Gain3 : Gain  Gain=100
  Hit Crossing : HitCross  ZeroCross=off
  MinMax : MinMax  Inputs=2
  Product1 : Product  RndMeth=Zero
  Product2 : Product  RndMeth=Zero
  Sw6 : Switch  Threshold=0.5  ZeroCross=off  SaturateOnIntegerOverflow=on  InputSameDT=on
  Tanh : Trigonometry  Operator=tanh
  Tanh1 : Trigonometry  Operator=tanh
  Friction_Torque : Outport
  reset velocity : Outport  Port=2
  wires:
  Torque/1 -> Gain1/1, Abs2/1
  Sw6/1 -> Friction_Torque/1
  Hit Crossing/1 -> reset velocity/1, Sw6/2
  Abs2/1 -> MinMax/2
  MinMax/1 -> Product2/1
  Product2/1 -> Sw6/1
  Product1/1 -> Sw6/3
  Gain2/1 -> MinMax/1
  velocity state/1 -> Hit Crossing/1
  Gain/1 -> Product1/1
  Gain1/1 -> Tanh/1
  Tanh/1 -> Product2/2
  Gain3/1 -> Tanh1/1
  Tanh1/1 -> Product1/2
  velocity/1 -> Gain3/1
  torque load value pod/1 -> Gain/1, Gain2/1

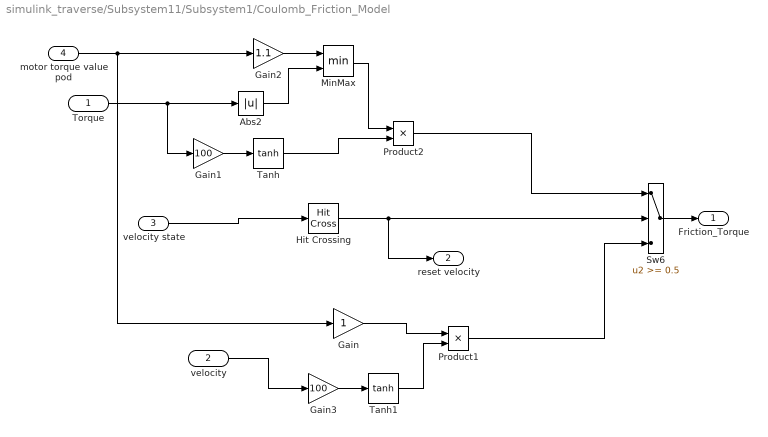
== system simulink_traverse/Subsystem11/Subsystem1/Coulomb_Friction_Model ==
  Torque : Inport
  velocity : Inport  Port=2
  velocity state : Inport  Port=3
  motor torque value pod : Inport  Port=4
  Abs2 : Abs  ZeroCross=off
  Gain : Gain
  Gain1 : Gain  Gain=100
  Gain2 : Gain  Gain=1.1
  Gain3 : Gain  Gain=100
  Hit Crossing : HitCross  ZeroCross=off
  MinMax : MinMax  Inputs=2
  Product1 : Product  RndMeth=Zero
  Product2 : Product  RndMeth=Zero
  Sw6 : Switch  Threshold=0.5  ZeroCross=off  SaturateOnIntegerOverflow=on  InputSameDT=on
  Tanh : Trigonometry  Operator=tanh
  Tanh1 : Trigonometry  Operator=tanh
  Friction_Torque : Outport
  reset velocity : Outport  Port=2
  wires:
  Torque/1 -> Gain1/1, Abs2/1
  Hit Crossing/1 -> reset velocity/1, Sw6/2
  Abs2/1 -> MinMax/2
  MinMax/1 -> Product2/1
  Product2/1 -> Sw6/1
  Product1/1 -> Sw6/3
  Gain2/1 -> MinMax/1
  velocity state/1 -> Hit Crossing/1
  Gain/1 -> Product1/1
  Gain1/1 -> Tanh/1
  Gain3/1 -> Tanh1/1
  Tanh/1 -> Product2/2
  Tanh1/1 -> Product1/2
  velocity/1 -> Gain3/1
  motor torque value pod/1 -> Gain2/1, Gain/1
  Sw6/1 -> Friction_Torque/1

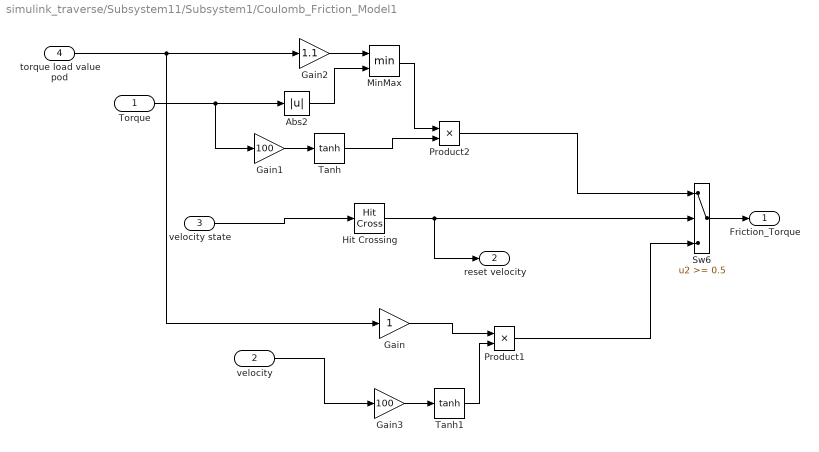
== system simulink_traverse/Subsystem11/Subsystem1/Coulomb_Friction_Model1 ==
  Torque : Inport
  velocity : Inport  Port=2
  velocity state : Inport  Port=3
  torque load value pod : Inport  Port=4
  Abs2 : Abs  ZeroCross=off
  Gain : Gain
  Gain1 : Gain  Gain=100
  Gain2 : Gain  Gain=1.1
  Gain3 : Gain  Gain=100
  Hit Crossing : HitCross  ZeroCross=off
  MinMax : MinMax  Inputs=2
  Product1 : Product  RndMeth=Zero
  Product2 : Product  RndMeth=Zero
  Sw6 : Switch  Threshold=0.5  ZeroCross=off  SaturateOnIntegerOverflow=on  InputSameDT=on
  Tanh : Trigonometry  Operator=tanh
  Tanh1 : Trigonometry  Operator=tanh
  Friction_Torque : Outport
  reset velocity : Outport  Port=2
  wires:
  Torque/1 -> Gain1/1, Abs2/1
  Sw6/1 -> Friction_Torque/1
  Hit Crossing/1 -> reset velocity/1, Sw6/2
  Abs2/1 -> MinMax/2
  MinMax/1 -> Product2/1
  Product2/1 -> Sw6/1
  Product1/1 -> Sw6/3
  Gain2/1 -> MinMax/1
  velocity state/1 -> Hit Crossing/1
  Gain/1 -> Product1/1
  Gain1/1 -> Tanh/1
  Tanh/1 -> Product2/2
  Gain3/1 -> Tanh1/1
  Tanh1/1 -> Product1/2
  velocity/1 -> Gain3/1
  torque load value pod/1 -> Gain/1, Gain2/1
